simulink model "pd_path_sg"  (R2013b)
settings: Solver=ode45  StartTime=0.0  StopTime=10  RelTol=1e-3
undefined symbols (not defined in the file or in its folder): A, A2, B, C, D, EVAL, i, output_samp_bcoef, PCIN, reg_pk_lim, reg_plim, reg_scale, reg_sr_lim, reg_staclr, reg_txgain, THIS_DATE, W, X, Z
undefined symbols (not defined in the file): lut_address, lut_address_s5, reg_dltap
libraries: xbsIndex_r4 x3819, lut_ram_vhdl x32
(part 27 of 31)

== system pd_path_sg/output_sw_B/config_regs1/perbus_reg3 ==
  addr : Inport
  din : Inport  Port=2
  we : Inport  Port=3
  rst : Inport  Port=4
  Logical1 : xbsIndex_r4/Logical  logical_function=AND  inputs=2  en=off  latency=0  precision=Full  arith_type=Unsigned  n_bits=16  bin_pt=0  align_bp=on  dbl_ovrd=off  block_type=logical
  REG_ADDR : xbsIndex_r4/Constant  const=reg_txgain(para_band+1)  gui_display_data_type=Fixed-point  arith_type=Unsigned  n_bits=12  bin_pt=0  preci_type=Single  exp_width=8  frac_width=24  explicit_period=off  period=1  equ=P=C  opselect=C  inp2=PCIN>>17  opr=+  inp1=P  carry=CIN  dbl_ovrd=off  block_type=constant
  Register : xbsIndex_r4/Register  init=16384  rst=on  en=on  dbl_ovrd=off  block_type=register
  Relational2 : xbsIndex_r4/Relational  mode=a=b  op_type=Bool  en=off  latency=0  dbl_ovrd=off  block_type=relational
  q : Outport
  wires:
  REG_ADDR/1 -> Relational2/2
  Relational2/1 -> Logical1/2
  Logical1/1 -> Register/3
  addr/1 -> Relational2/1
  we/1 -> Logical1/1
  din/1 -> Register/1
  Register/1 -> q/1
  rst/1 -> Register/2

== system pd_path_sg/output_sw_B/detect_i/cut8bit ==
  d : Inport
  Convert : xbsIndex_r4/Convert  gui_display_data_type=Fixed-point  arith_type="Signed  (2's comp)"  n_bits=17  bin_pt=0  float_type=Single  exp_bits=8  fraction_bits=24  quantization=Truncate  overflow=Wrap  en=off  latency=0  pipeline=off  dbl_ovrd=off  block_type=convert
  Reinterpret4 : xbsIndex_r4/Reinterpret  force_arith_type=on  arith_type="Signed  (2's comp)"  force_bin_pt=off  bin_pt=0  block_type=reinterpret
  Slice1 : xbsIndex_r4/Slice  nbits=9  boolean_output=off  mode=Upper Bit Location + Width  bit1=0  base1=MSB of Input  bit0=0  base0=LSB of Input  dbl_ovrd=off  block_type=slice
  q : Outport
  wires:
  Reinterpret4/1 -> q/1
  d/1 -> Convert/1
  Convert/1 -> Slice1/1
  Slice1/1 -> Reinterpret4/1

== system pd_path_sg/output_sw_B/detect_i/cut8bit1 ==
  d : Inport
  Convert : xbsIndex_r4/Convert  gui_display_data_type=Fixed-point  arith_type="Signed  (2's comp)"  n_bits=17  bin_pt=0  float_type=Single  exp_bits=8  fraction_bits=24  quantization=Truncate  overflow=Wrap  en=off  latency=0  pipeline=off  dbl_ovrd=off  block_type=convert
  Reinterpret4 : xbsIndex_r4/Reinterpret  force_arith_type=on  arith_type="Signed  (2's comp)"  force_bin_pt=off  bin_pt=0  block_type=reinterpret
  Slice1 : xbsIndex_r4/Slice  nbits=9  boolean_output=off  mode=Upper Bit Location + Width  bit1=0  base1=MSB of Input  bit0=0  base0=LSB of Input  dbl_ovrd=off  block_type=slice
  q : Outport
  wires:
  Slice1/1 -> Reinterpret4/1
  Convert/1 -> Slice1/1
  d/1 -> Convert/1
  Reinterpret4/1 -> q/1

== system pd_path_sg/output_sw_B/detect_i/cut8bit2 ==
  d : Inport
  Convert : xbsIndex_r4/Convert  gui_display_data_type=Fixed-point  arith_type="Signed  (2's comp)"  n_bits=17  bin_pt=0  float_type=Single  exp_bits=8  fraction_bits=24  quantization=Truncate  overflow=Wrap  en=off  latency=0  pipeline=off  dbl_ovrd=off  block_type=convert
  Reinterpret4 : xbsIndex_r4/Reinterpret  force_arith_type=on  arith_type="Signed  (2's comp)"  force_bin_pt=off  bin_pt=0  block_type=reinterpret
  Slice1 : xbsIndex_r4/Slice  nbits=9  boolean_output=off  mode=Upper Bit Location + Width  bit1=0  base1=MSB of Input  bit0=0  base0=LSB of Input  dbl_ovrd=off  block_type=slice
  q : Outport
  wires:
  Reinterpret4/1 -> q/1
  d/1 -> Convert/1
  Convert/1 -> Slice1/1
  Slice1/1 -> Reinterpret4/1

== system pd_path_sg/output_sw_B/detect_i/cut8bit3 ==
  d : Inport
  Convert : xbsIndex_r4/Convert  gui_display_data_type=Fixed-point  arith_type="Signed  (2's comp)"  n_bits=17  bin_pt=0  float_type=Single  exp_bits=8  fraction_bits=24  quantization=Truncate  overflow=Wrap  en=off  latency=0  pipeline=off  dbl_ovrd=off  block_type=convert
  Reinterpret4 : xbsIndex_r4/Reinterpret  force_arith_type=on  arith_type="Signed  (2's comp)"  force_bin_pt=off  bin_pt=0  block_type=reinterpret
  Slice1 : xbsIndex_r4/Slice  nbits=9  boolean_output=off  mode=Upper Bit Location + Width  bit1=0  base1=MSB of Input  bit0=0  base0=LSB of Input  dbl_ovrd=off  block_type=slice
  q : Outport
  wires:
  Slice1/1 -> Reinterpret4/1
  Convert/1 -> Slice1/1
  d/1 -> Convert/1
  Reinterpret4/1 -> q/1

== system pd_path_sg/output_sw_B/detect_i/cut8bit4 ==
  d : Inport
  Convert : xbsIndex_r4/Convert  gui_display_data_type=Fixed-point  arith_type="Signed  (2's comp)"  n_bits=17  bin_pt=0  float_type=Single  exp_bits=8  fraction_bits=24  quantization=Truncate  overflow=Wrap  en=off  latency=0  pipeline=off  dbl_ovrd=off  block_type=convert
  Reinterpret4 : xbsIndex_r4/Reinterpret  force_arith_type=on  arith_type="Signed  (2's comp)"  force_bin_pt=off  bin_pt=0  block_type=reinterpret
  Slice1 : xbsIndex_r4/Slice  nbits=9  boolean_output=off  mode=Upper Bit Location + Width  bit1=0  base1=MSB of Input  bit0=0  base0=LSB of Input  dbl_ovrd=off  block_type=slice
  q : Outport
  wires:
  Reinterpret4/1 -> q/1
  d/1 -> Convert/1
  Convert/1 -> Slice1/1
  Slice1/1 -> Reinterpret4/1

== system pd_path_sg/output_sw_B/detect_i/cut8bit5 ==
  d : Inport
  Convert : xbsIndex_r4/Convert  gui_display_data_type=Fixed-point  arith_type="Signed  (2's comp)"  n_bits=17  bin_pt=0  float_type=Single  exp_bits=8  fraction_bits=24  quantization=Truncate  overflow=Wrap  en=off  latency=0  pipeline=off  dbl_ovrd=off  block_type=convert
  Reinterpret4 : xbsIndex_r4/Reinterpret  force_arith_type=on  arith_type="Signed  (2's comp)"  force_bin_pt=off  bin_pt=0  block_type=reinterpret
  Slice1 : xbsIndex_r4/Slice  nbits=9  boolean_output=off  mode=Upper Bit Location + Width  bit1=0  base1=MSB of Input  bit0=0  base0=LSB of Input  dbl_ovrd=off  block_type=slice
  q : Outport
  wires:
  Slice1/1 -> Reinterpret4/1
  Convert/1 -> Slice1/1
  d/1 -> Convert/1
  Reinterpret4/1 -> q/1

== system pd_path_sg/output_sw_B/detect_q/cut8bit ==
  d : Inport
  Convert : xbsIndex_r4/Convert  gui_display_data_type=Fixed-point  arith_type="Signed  (2's comp)"  n_bits=17  bin_pt=0  float_type=Single  exp_bits=8  fraction_bits=24  quantization=Truncate  overflow=Wrap  en=off  latency=0  pipeline=off  dbl_ovrd=off  block_type=convert
  Reinterpret4 : xbsIndex_r4/Reinterpret  force_arith_type=on  arith_type="Signed  (2's comp)"  force_bin_pt=off  bin_pt=0  block_type=reinterpret
  Slice1 : xbsIndex_r4/Slice  nbits=9  boolean_output=off  mode=Upper Bit Location + Width  bit1=0  base1=MSB of Input  bit0=0  base0=LSB of Input  dbl_ovrd=off  block_type=slice
  q : Outport
  wires:
  Slice1/1 -> Reinterpret4/1
  Convert/1 -> Slice1/1
  d/1 -> Convert/1
  Reinterpret4/1 -> q/1

== system pd_path_sg/output_sw_B/detect_q/cut8bit1 ==
  d : Inport
  Convert : xbsIndex_r4/Convert  gui_display_data_type=Fixed-point  arith_type="Signed  (2's comp)"  n_bits=17  bin_pt=0  float_type=Single  exp_bits=8  fraction_bits=24  quantization=Truncate  overflow=Wrap  en=off  latency=0  pipeline=off  dbl_ovrd=off  block_type=convert
  Reinterpret4 : xbsIndex_r4/Reinterpret  force_arith_type=on  arith_type="Signed  (2's comp)"  force_bin_pt=off  bin_pt=0  block_type=reinterpret
  Slice1 : xbsIndex_r4/Slice  nbits=9  boolean_output=off  mode=Upper Bit Location + Width  bit1=0  base1=MSB of Input  bit0=0  base0=LSB of Input  dbl_ovrd=off  block_type=slice
  q : Outport
  wires:
  Reinterpret4/1 -> q/1
  d/1 -> Convert/1
  Convert/1 -> Slice1/1
  Slice1/1 -> Reinterpret4/1

== system pd_path_sg/output_sw_B/detect_q/cut8bit2 ==
  d : Inport
  Convert : xbsIndex_r4/Convert  gui_display_data_type=Fixed-point  arith_type="Signed  (2's comp)"  n_bits=17  bin_pt=0  float_type=Single  exp_bits=8  fraction_bits=24  quantization=Truncate  overflow=Wrap  en=off  latency=0  pipeline=off  dbl_ovrd=off  block_type=convert
  Reinterpret4 : xbsIndex_r4/Reinterpret  force_arith_type=on  arith_type="Signed  (2's comp)"  force_bin_pt=off  bin_pt=0  block_type=reinterpret
  Slice1 : xbsIndex_r4/Slice  nbits=9  boolean_output=off  mode=Upper Bit Location + Width  bit1=0  base1=MSB of Input  bit0=0  base0=LSB of Input  dbl_ovrd=off  block_type=slice
  q : Outport
  wires:
  Slice1/1 -> Reinterpret4/1
  Convert/1 -> Slice1/1
  d/1 -> Convert/1
  Reinterpret4/1 -> q/1

== system pd_path_sg/output_sw_B/detect_q/cut8bit3 ==
  d : Inport
  Convert : xbsIndex_r4/Convert  gui_display_data_type=Fixed-point  arith_type="Signed  (2's comp)"  n_bits=17  bin_pt=0  float_type=Single  exp_bits=8  fraction_bits=24  quantization=Truncate  overflow=Wrap  en=off  latency=0  pipeline=off  dbl_ovrd=off  block_type=convert
  Reinterpret4 : xbsIndex_r4/Reinterpret  force_arith_type=on  arith_type="Signed  (2's comp)"  force_bin_pt=off  bin_pt=0  block_type=reinterpret
  Slice1 : xbsIndex_r4/Slice  nbits=9  boolean_output=off  mode=Upper Bit Location + Width  bit1=0  base1=MSB of Input  bit0=0  base0=LSB of Input  dbl_ovrd=off  block_type=slice
  q : Outport
  wires:
  Reinterpret4/1 -> q/1
  d/1 -> Convert/1
  Convert/1 -> Slice1/1
  Slice1/1 -> Reinterpret4/1

== system pd_path_sg/output_sw_B/detect_q/cut8bit4 ==
  d : Inport
  Convert : xbsIndex_r4/Convert  gui_display_data_type=Fixed-point  arith_type="Signed  (2's comp)"  n_bits=17  bin_pt=0  float_type=Single  exp_bits=8  fraction_bits=24  quantization=Truncate  overflow=Wrap  en=off  latency=0  pipeline=off  dbl_ovrd=off  block_type=convert
  Reinterpret4 : xbsIndex_r4/Reinterpret  force_arith_type=on  arith_type="Signed  (2's comp)"  force_bin_pt=off  bin_pt=0  block_type=reinterpret
  Slice1 : xbsIndex_r4/Slice  nbits=9  boolean_output=off  mode=Upper Bit Location + Width  bit1=0  base1=MSB of Input  bit0=0  base0=LSB of Input  dbl_ovrd=off  block_type=slice
  q : Outport
  wires:
  Slice1/1 -> Reinterpret4/1
  Convert/1 -> Slice1/1
  d/1 -> Convert/1
  Reinterpret4/1 -> q/1

== system pd_path_sg/output_sw_B/detect_q/cut8bit5 ==
  d : Inport
  Convert : xbsIndex_r4/Convert  gui_display_data_type=Fixed-point  arith_type="Signed  (2's comp)"  n_bits=17  bin_pt=0  float_type=Single  exp_bits=8  fraction_bits=24  quantization=Truncate  overflow=Wrap  en=off  latency=0  pipeline=off  dbl_ovrd=off  block_type=convert
  Reinterpret4 : xbsIndex_r4/Reinterpret  force_arith_type=on  arith_type="Signed  (2's comp)"  force_bin_pt=off  bin_pt=0  block_type=reinterpret
  Slice1 : xbsIndex_r4/Slice  nbits=9  boolean_output=off  mode=Upper Bit Location + Width  bit1=0  base1=MSB of Input  bit0=0  base0=LSB of Input  dbl_ovrd=off  block_type=slice
  q : Outport
  wires:
  Reinterpret4/1 -> q/1
  d/1 -> Convert/1
  Convert/1 -> Slice1/1
  Slice1/1 -> Reinterpret4/1

== system pd_path_sg/resamp_mod/mod0/imag_modu ==
  Ai : Inport
  Aq : Inport  Port=2
  Bi : Inport  Port=3
  Bq : Inport  Port=4
  sin : Inport  Port=5
  cos : Inport  Port=6
  Constant1 : xbsIndex_r4/Constant  const=2^13  gui_display_data_type=Fixed-point  arith_type=Signed (2's comp)  n_bits=48  bin_pt=0  preci_type=Single  exp_width=8  frac_width=24  explicit_period=off  period=1  equ=P=C  opselect=C  inp2=PCIN>>17  opr=+  inp1=P  carry=CIN  dbl_ovrd=off  block_type=constant
  Convert10 : xbsIndex_r4/Convert  gui_display_data_type=Fixed-point  arith_type="Signed  (2's comp)"  n_bits=18  bin_pt=0  float_type=Single  exp_bits=8  fraction_bits=24  quantization=Truncate  overflow=Wrap  en=off  latency=0  pipeline=off  dbl_ovrd=off  block_type=convert
  Convert11 : xbsIndex_r4/Convert  gui_display_data_type=Fixed-point  arith_type="Signed  (2's comp)"  n_bits=27  bin_pt=0  float_type=Single  exp_bits=8  fraction_bits=24  quantization=Truncate  overflow=Wrap  en=off  latency=0  pipeline=off  dbl_ovrd=off  block_type=convert
  Convert5 : xbsIndex_r4/Convert  gui_display_data_type=Fixed-point  arith_type="Signed  (2's comp)"  n_bits=30  bin_pt=0  float_type=Single  exp_bits=8  fraction_bits=24  quantization=Truncate  overflow=Wrap  en=off  latency=0  pipeline=off  dbl_ovrd=off  block_type=convert
  Convert6 : xbsIndex_r4/Convert  gui_display_data_type=Fixed-point  arith_type="Signed  (2's comp)"  n_bits=18  bin_pt=0  float_type=Single  exp_bits=8  fraction_bits=24  quantization=Truncate  overflow=Wrap  en=off  latency=0  pipeline=off  dbl_ovrd=off  block_type=convert
  Convert8 : xbsIndex_r4/Convert  gui_display_data_type=Fixed-point  arith_type="Signed  (2's comp)"  n_bits=27  bin_pt=0  float_type=Single  exp_bits=8  fraction_bits=24  quantization=Truncate  overflow=Wrap  en=off  latency=0  pipeline=off  dbl_ovrd=off  block_type=convert
  Convert9 : xbsIndex_r4/Convert  gui_display_data_type=Fixed-point  arith_type="Signed  (2's comp)"  n_bits=30  bin_pt=0  float_type=Single  exp_bits=8  fraction_bits=24  quantization=Truncate  overflow=Wrap  en=off  latency=0  pipeline=off  dbl_ovrd=off  block_type=convert
  "DSP48E2 " : xbsIndex_r4/DSP48E2   use_a=Direct from A Port  use_b=Direct from B Port  addsub_mode=ONE48  xl_useadderonly=off  xl_dynamicmult=off  preaddinsel=A  amultsel=AD  bmultsel=B  enable_d=on  reset_preg=off  auto_reset_pr=RESET  pattern_from_creg=1  pattern='000000000000'  mask_from_creg=1  pattern_mask='000000000000'  rnd='000000000000'  widexor=off  xormode=1  use_op=on  use_creg=on  rst_all=off  en_all=off  use_pcin=off  use_carrycascin=off  use_multsignin=off  use_carryout=off  use_patterndetect=off  use_patternbdetect=off  use_overflow=off  use_underflow=off  use_acout=off  use_bcout=off  use_pcout=on  use_multsignout=off  use_carrycascout=off  pipeline_a=1  pipeline_b=2  pipeline_acout=1  pipeline_bcout=1  pipeline_c=on  pipeline_p=on  pipeline_mult=on  pipeline_opmode=on  pipeline_alumode=on  pipeline_carryin=on  pipeline_carryinsel=on  dreg=on  adreg=on  register_inmode=on  rst_a=off  rst_b=off  rst_c=off  rst_mult=off  rst_p=off  rst_carry_in=off  rst_alumode=off  rst_ctrl=off  reset_port_d=off  reset_port_inmode=off  en_a1=off  en_a2=off  en_b1=off  en_b2=off  en_c=off  en_mult=off  en_p=off  en_carry_in=off  en_alumode=off  en_multcarryin=off  en_ctrl=off  enable_port_regd=off  enable_port_regad=off  enable_port_reginmode=off  alumode_inverted=off  alumode_inverted_value='0000'  is_carryin_inverted=off  inmode_inverted=off  inmode_inverted_value='00000'  opmode_inverted=off  opmode_inverted_value='000000000'  is_rstallcarryin_inverted=off  is_rstalumode_inverted=off  is_rsta_inverted=off  is_rstb_inverted=off  is_rstc_inverted=off  is_rstd_inverted=off  is_rstctrl_inverted=off  is_rstinmode_inverted=off  is_rstm_inverted=off  is_rstp_inverted=off  use_synth_model=off  is_clk_inverted=false  block_type=dsp48e2
  DSP48E2 1 : xbsIndex_r4/DSP48E2   use_a=Direct from A Port  use_b=Direct from B Port  addsub_mode=ONE48  xl_useadderonly=off  xl_dynamicmult=off  preaddinsel=A  amultsel=AD  bmultsel=B  enable_d=on  reset_preg=off  auto_reset_pr=RESET  pattern_from_creg=1  pattern='000000000000'  mask_from_creg=1  pattern_mask='000000000000'  rnd='000000000000'  widexor=off  xormode=1  use_op=on  use_creg=off  rst_all=off  en_all=off  use_pcin=on  use_carrycascin=off  use_multsignin=off  use_carryout=off  use_patterndetect=off  use_patternbdetect=off  use_overflow=off  use_underflow=off  use_acout=off  use_bcout=off  use_pcout=off  use_multsignout=off  use_carrycascout=off  pipeline_a=2  pipeline_b=2  pipeline_acout=1  pipeline_bcout=1  pipeline_c=on  pipeline_p=on  pipeline_mult=on  pipeline_opmode=on  pipeline_alumode=on  pipeline_carryin=on  pipeline_carryinsel=on  dreg=on  adreg=on  register_inmode=on  rst_a=off  rst_b=off  rst_c=off  rst_mult=off  rst_p=off  rst_carry_in=off  rst_alumode=off  rst_ctrl=off  reset_port_d=off  reset_port_inmode=off  en_a1=off  en_a2=off  en_b1=off  en_b2=off  en_c=off  en_mult=off  en_p=off  en_carry_in=off  en_alumode=off  en_multcarryin=off  en_ctrl=off  enable_port_regd=off  enable_port_regad=off  enable_port_reginmode=off  alumode_inverted=off  alumode_inverted_value='0000'  is_carryin_inverted=off  inmode_inverted=off  inmode_inverted_value='00000'  opmode_inverted=off  opmode_inverted_value='000000000'  is_rstallcarryin_inverted=off  is_rstalumode_inverted=off  is_rsta_inverted=off  is_rstb_inverted=off  is_rstc_inverted=off  is_rstd_inverted=off  is_rstctrl_inverted=off  is_rstinmode_inverted=off  is_rstm_inverted=off  is_rstp_inverted=off  use_synth_model=off  is_clk_inverted=false  block_type=dsp48e2
  Delay : xbsIndex_r4/Delay  rst=off  infoeditControl=Selection of Reset will increase slice count due to use of real FFs and instead of SRLs  en=off  latency=1  reg_retiming=off  dbl_ovrd=off  block_type=delay
      settings: infoedit=Hardware notes: A delay line is a chain, each link of which is an SRL16 or SRL32 followed by a flip-flop.
  Delay1 : xbsIndex_r4/Delay  rst=off  infoeditControl=Selection of Reset will increase slice count due to use of real FFs and instead of SRLs  en=off  latency=1  reg_retiming=off  dbl_ovrd=off  block_type=delay
      settings: infoedit=Hardware notes: A delay line is a chain, each link of which is an SRL16 or SRL32 followed by a flip-flop.
  Opmode1 : xbsIndex_r4/Opmode  device=DSP48E2  equ=P=C+(A*B)  operation=Custom  inmode_0_3=D+A2  inmode_1_3=(D+A)*B  preaddinsel=A  amultsel=AD  bmultsel=B  inmode_0=A2  inmode_4=B2  logicinstr=X + W + Z  z_mux=C  xy_mux=A*B  w_mux=0  carry=0  dbl_ovrd=off  operand=+  x_mux=P  block_type=opmode
  Opmode4 : xbsIndex_r4/Opmode  device=DSP48E2  equ=P=PCIN+(A*B)  operation=Custom  inmode_0_3=D+A2  inmode_1_3=(D-A)*B  preaddinsel=A  amultsel=AD  bmultsel=B  inmode_0=A2  inmode_4=B2  logicinstr=X + W + Z  z_mux=PCIN  xy_mux=A*B  w_mux=0  carry=0  dbl_ovrd=off  operand=+  x_mux=P  block_type=opmode
  Reinterpret{5..10,13} (7 alike) : xbsIndex_r4/Reinterpret  force_arith_type=on  arith_type="Signed  (2's comp)"  force_bin_pt=on  bin_pt=0  block_type=reinterpret
  Terminator1 : Terminator
  round1 : Subsystem
  out_imag : Outport
  wires:
  Convert11/1 -> Delay/1
  Convert10/1 -> Delay1/1
  Reinterpret9/1 -> Convert10/1
  Reinterpret10/1 -> Convert11/1
  Reinterpret8/1 -> Convert9/1
  Constant1/1 -> "DSP48E2 "/3
  Bq/1 -> Reinterpret7/1
  Convert9/1 -> DSP48E2 1/1
  sin/1 -> Reinterpret9/1
  Reinterpret7/1 -> Convert8/1
  Aq/1 -> Reinterpret5/1
  cos/1 -> Reinterpret6/1
  Convert6/1 -> "DSP48E2 "/2
  Convert8/1 -> "DSP48E2 "/4
  Ai/1 -> Reinterpret10/1
  Bi/1 -> Reinterpret8/1
  "DSP48E2 "/1 -> Terminator1/1
  DSP48E2 1/1 -> Reinterpret13/1
  Convert5/1 -> "DSP48E2 "/1
  Reinterpret6/1 -> Convert6/1
  "DSP48E2 "/2 -> DSP48E2 1/3
  Reinterpret5/1 -> Convert5/1
  Reinterpret13/1 -> round1/1(d)
  round1/1(q) -> out_imag/1
  Delay/1 -> DSP48E2 1/4
  Delay1/1 -> DSP48E2 1/2
  Opmode1/1 -> "DSP48E2 "/5
  Opmode4/1 -> DSP48E2 1/5

== system pd_path_sg/resamp_mod/mod0/real_modu ==
  Ai : Inport
  Aq : Inport  Port=2
  Bi : Inport  Port=3
  Bq : Inport  Port=4
  sin : Inport  Port=5
  cos : Inport  Port=6
  Constant3 : xbsIndex_r4/Constant  const=2^13  gui_display_data_type=Fixed-point  arith_type=Signed (2's comp)  n_bits=48  bin_pt=0  preci_type=Single  exp_width=8  frac_width=24  explicit_period=off  period=1  equ=P=C  opselect=C  inp2=PCIN>>17  opr=+  inp1=P  carry=CIN  dbl_ovrd=off  block_type=constant
  Convert : xbsIndex_r4/Convert  gui_display_data_type=Fixed-point  arith_type="Signed  (2's comp)"  n_bits=30  bin_pt=0  float_type=Single  exp_bits=8  fraction_bits=24  quantization=Truncate  overflow=Wrap  en=off  latency=0  pipeline=off  dbl_ovrd=off  block_type=convert
  Convert1 : xbsIndex_r4/Convert  gui_display_data_type=Fixed-point  arith_type="Signed  (2's comp)"  n_bits=18  bin_pt=0  float_type=Single  exp_bits=8  fraction_bits=24  quantization=Truncate  overflow=Wrap  en=off  latency=0  pipeline=off  dbl_ovrd=off  block_type=convert
  Convert2 : xbsIndex_r4/Convert  gui_display_data_type=Fixed-point  arith_type="Signed  (2's comp)"  n_bits=18  bin_pt=0  float_type=Single  exp_bits=8  fraction_bits=24  quantization=Truncate  overflow=Wrap  en=off  latency=0  pipeline=off  dbl_ovrd=off  block_type=convert
  Convert3 : xbsIndex_r4/Convert  gui_display_data_type=Fixed-point  arith_type="Signed  (2's comp)"  n_bits=30  bin_pt=0  float_type=Single  exp_bits=8  fraction_bits=24  quantization=Truncate  overflow=Wrap  en=off  latency=0  pipeline=off  dbl_ovrd=off  block_type=convert
  Convert4 : xbsIndex_r4/Convert  gui_display_data_type=Fixed-point  arith_type="Signed  (2's comp)"  n_bits=27  bin_pt=0  float_type=Single  exp_bits=8  fraction_bits=24  quantization=Truncate  overflow=Wrap  en=off  latency=0  pipeline=off  dbl_ovrd=off  block_type=convert
  Convert7 : xbsIndex_r4/Convert  gui_display_data_type=Fixed-point  arith_type="Signed  (2's comp)"  n_bits=27  bin_pt=0  float_type=Single  exp_bits=8  fraction_bits=24  quantization=Truncate  overflow=Wrap  en=off  latency=0  pipeline=off  dbl_ovrd=off  block_type=convert
  "DSP48E2 " : xbsIndex_r4/DSP48E2   use_a=Direct from A Port  use_b=Direct from B Port  addsub_mode=ONE48  xl_useadderonly=off  xl_dynamicmult=off  preaddinsel=A  amultsel=AD  bmultsel=B  enable_d=on  reset_preg=off  auto_reset_pr=RESET  pattern_from_creg=1  pattern='000000000000'  mask_from_creg=1  pattern_mask='000000000000'  rnd='000000000000'  widexor=off  xormode=1  use_op=on  use_creg=on  rst_all=off  en_all=off  use_pcin=off  use_carrycascin=off  use_multsignin=off  use_carryout=off  use_patterndetect=off  use_patternbdetect=off  use_overflow=off  use_underflow=off  use_acout=off  use_bcout=off  use_pcout=on  use_multsignout=off  use_carrycascout=off  pipeline_a=1  pipeline_b=2  pipeline_acout=1  pipeline_bcout=1  pipeline_c=on  pipeline_p=on  pipeline_mult=on  pipeline_opmode=on  pipeline_alumode=on  pipeline_carryin=on  pipeline_carryinsel=on  dreg=on  adreg=on  register_inmode=on  rst_a=off  rst_b=off  rst_c=off  rst_mult=off  rst_p=off  rst_carry_in=off  rst_alumode=off  rst_ctrl=off  reset_port_d=off  reset_port_inmode=off  en_a1=off  en_a2=off  en_b1=off  en_b2=off  en_c=off  en_mult=off  en_p=off  en_carry_in=off  en_alumode=off  en_multcarryin=off  en_ctrl=off  enable_port_regd=off  enable_port_regad=off  enable_port_reginmode=off  alumode_inverted=off  alumode_inverted_value='0000'  is_carryin_inverted=off  inmode_inverted=off  inmode_inverted_value='00000'  opmode_inverted=off  opmode_inverted_value='000000000'  is_rstallcarryin_inverted=off  is_rstalumode_inverted=off  is_rsta_inverted=off  is_rstb_inverted=off  is_rstc_inverted=off  is_rstd_inverted=off  is_rstctrl_inverted=off  is_rstinmode_inverted=off  is_rstm_inverted=off  is_rstp_inverted=off  use_synth_model=off  is_clk_inverted=false  block_type=dsp48e2
  DSP48E2 1 : xbsIndex_r4/DSP48E2   use_a=Direct from A Port  use_b=Direct from B Port  addsub_mode=ONE48  xl_useadderonly=off  xl_dynamicmult=off  preaddinsel=A  amultsel=AD  bmultsel=B  enable_d=on  reset_preg=off  auto_reset_pr=RESET  pattern_from_creg=1  pattern='000000000000'  mask_from_creg=1  pattern_mask='000000000000'  rnd='000000000000'  widexor=off  xormode=1  use_op=on  use_creg=off  rst_all=off  en_all=off  use_pcin=on  use_carrycascin=off  use_multsignin=off  use_carryout=off  use_patterndetect=off  use_patternbdetect=off  use_overflow=off  use_underflow=off  use_acout=off  use_bcout=off  use_pcout=off  use_multsignout=off  use_carrycascout=off  pipeline_a=2  pipeline_b=2  pipeline_acout=1  pipeline_bcout=1  pipeline_c=on  pipeline_p=on  pipeline_mult=on  pipeline_opmode=on  pipeline_alumode=on  pipeline_carryin=on  pipeline_carryinsel=on  dreg=on  adreg=on  register_inmode=on  rst_a=off  rst_b=off  rst_c=off  rst_mult=off  rst_p=off  rst_carry_in=off  rst_alumode=off  rst_ctrl=off  reset_port_d=off  reset_port_inmode=off  en_a1=off  en_a2=off  en_b1=off  en_b2=off  en_c=off  en_mult=off  en_p=off  en_carry_in=off  en_alumode=off  en_multcarryin=off  en_ctrl=off  enable_port_regd=off  enable_port_regad=off  enable_port_reginmode=off  alumode_inverted=off  alumode_inverted_value='0000'  is_carryin_inverted=off  inmode_inverted=off  inmode_inverted_value='00000'  opmode_inverted=off  opmode_inverted_value='000000000'  is_rstallcarryin_inverted=off  is_rstalumode_inverted=off  is_rsta_inverted=off  is_rstb_inverted=off  is_rstc_inverted=off  is_rstd_inverted=off  is_rstctrl_inverted=off  is_rstinmode_inverted=off  is_rstm_inverted=off  is_rstp_inverted=off  use_synth_model=off  is_clk_inverted=false  block_type=dsp48e2
  Delay : xbsIndex_r4/Delay  rst=off  infoeditControl=Selection of Reset will increase slice count due to use of real FFs and instead of SRLs  en=off  latency=1  reg_retiming=off  dbl_ovrd=off  block_type=delay
      settings: infoedit=Hardware notes: A delay line is a chain, each link of which is an SRL16 or SRL32 followed by a flip-flop.
  Delay1 : xbsIndex_r4/Delay  rst=off  infoeditControl=Selection of Reset will increase slice count due to use of real FFs and instead of SRLs  en=off  latency=1  reg_retiming=off  dbl_ovrd=off  block_type=delay
      settings: infoedit=Hardware notes: A delay line is a chain, each link of which is an SRL16 or SRL32 followed by a flip-flop.
  Opmode2 : xbsIndex_r4/Opmode  device=DSP48E2  equ=P=C+(A*B)  operation=Custom  inmode_0_3=D+A2  inmode_1_3=(D+A)*B  preaddinsel=A  amultsel=AD  bmultsel=B  inmode_0=A2  inmode_4=B2  logicinstr=X + W + Z  z_mux=C  xy_mux=A*B  w_mux=0  carry=0  dbl_ovrd=off  operand=+  x_mux=P  block_type=opmode
  Opmode3 : xbsIndex_r4/Opmode  device=DSP48E2  equ=P=PCIN+(A*B)  operation=Custom  inmode_0_3=D+A2  inmode_1_3=(D-A)*B  preaddinsel=A  amultsel=AD  bmultsel=B  inmode_0=A2  inmode_4=B2  logicinstr=X + W + Z  z_mux=PCIN  xy_mux=A*B  w_mux=0  carry=0  dbl_ovrd=off  operand=+  x_mux=P  block_type=opmode
  Reinterpret{,1..4,11,13} (7 alike) : xbsIndex_r4/Reinterpret  force_arith_type=on  arith_type="Signed  (2's comp)"  force_bin_pt=on  bin_pt=0  block_type=reinterpret
  Terminator : Terminator
  round1 : Subsystem
  out_real : Outport
  wires:
  sin/1 -> Reinterpret1/1
  Aq/1 -> Reinterpret2/1
  Ai/1 -> Reinterpret4/1
  Bq/1 -> Reinterpret3/1
  cos/1 -> Reinterpret/1
  Bi/1 -> Reinterpret11/1
  "DSP48E2 "/2 -> DSP48E2 1/3
  "DSP48E2 "/1 -> Terminator/1
  DSP48E2 1/1 -> Reinterpret13/1
  Reinterpret4/1 -> Convert/1
  Convert1/1 -> "DSP48E2 "/2
  Convert/1 -> "DSP48E2 "/1
  Reinterpret/1 -> Convert1/1
  Convert4/1 -> Delay/1
  Convert2/1 -> Delay1/1
  Convert3/1 -> DSP48E2 1/1
  Reinterpret3/1 -> Convert4/1
  Reinterpret11/1 -> Convert7/1
  Constant3/1 -> "DSP48E2 "/3
  Reinterpret1/1 -> Convert2/1
  Convert7/1 -> "DSP48E2 "/4
  Reinterpret2/1 -> Convert3/1
  Reinterpret13/1 -> round1/1(d)
  round1/1(q) -> out_real/1
  Delay/1 -> DSP48E2 1/4
  Delay1/1 -> DSP48E2 1/2
  Opmode2/1 -> "DSP48E2 "/5
  Opmode3/1 -> DSP48E2 1/5

== system pd_path_sg/resamp_mod/mod1/imag_modu ==
  Ai : Inport
  Aq : Inport  Port=2
  Bi : Inport  Port=3
  Bq : Inport  Port=4
  sin : Inport  Port=5
  cos : Inport  Port=6
  Constant1 : xbsIndex_r4/Constant  const=2^13  gui_display_data_type=Fixed-point  arith_type=Signed (2's comp)  n_bits=48  bin_pt=0  preci_type=Single  exp_width=8  frac_width=24  explicit_period=off  period=1  equ=P=C  opselect=C  inp2=PCIN>>17  opr=+  inp1=P  carry=CIN  dbl_ovrd=off  block_type=constant
  Convert10 : xbsIndex_r4/Convert  gui_display_data_type=Fixed-point  arith_type="Signed  (2's comp)"  n_bits=18  bin_pt=0  float_type=Single  exp_bits=8  fraction_bits=24  quantization=Truncate  overflow=Wrap  en=off  latency=0  pipeline=off  dbl_ovrd=off  block_type=convert
  Convert11 : xbsIndex_r4/Convert  gui_display_data_type=Fixed-point  arith_type="Signed  (2's comp)"  n_bits=27  bin_pt=0  float_type=Single  exp_bits=8  fraction_bits=24  quantization=Truncate  overflow=Wrap  en=off  latency=0  pipeline=off  dbl_ovrd=off  block_type=convert
  Convert5 : xbsIndex_r4/Convert  gui_display_data_type=Fixed-point  arith_type="Signed  (2's comp)"  n_bits=30  bin_pt=0  float_type=Single  exp_bits=8  fraction_bits=24  quantization=Truncate  overflow=Wrap  en=off  latency=0  pipeline=off  dbl_ovrd=off  block_type=convert
  Convert6 : xbsIndex_r4/Convert  gui_display_data_type=Fixed-point  arith_type="Signed  (2's comp)"  n_bits=18  bin_pt=0  float_type=Single  exp_bits=8  fraction_bits=24  quantization=Truncate  overflow=Wrap  en=off  latency=0  pipeline=off  dbl_ovrd=off  block_type=convert
  Convert8 : xbsIndex_r4/Convert  gui_display_data_type=Fixed-point  arith_type="Signed  (2's comp)"  n_bits=27  bin_pt=0  float_type=Single  exp_bits=8  fraction_bits=24  quantization=Truncate  overflow=Wrap  en=off  latency=0  pipeline=off  dbl_ovrd=off  block_type=convert
  Convert9 : xbsIndex_r4/Convert  gui_display_data_type=Fixed-point  arith_type="Signed  (2's comp)"  n_bits=30  bin_pt=0  float_type=Single  exp_bits=8  fraction_bits=24  quantization=Truncate  overflow=Wrap  en=off  latency=0  pipeline=off  dbl_ovrd=off  block_type=convert
  "DSP48E2 " : xbsIndex_r4/DSP48E2   use_a=Direct from A Port  use_b=Direct from B Port  addsub_mode=ONE48  xl_useadderonly=off  xl_dynamicmult=off  preaddinsel=A  amultsel=AD  bmultsel=B  enable_d=on  reset_preg=off  auto_reset_pr=RESET  pattern_from_creg=1  pattern='000000000000'  mask_from_creg=1  pattern_mask='000000000000'  rnd='000000000000'  widexor=off  xormode=1  use_op=on  use_creg=on  rst_all=off  en_all=off  use_pcin=off  use_carrycascin=off  use_multsignin=off  use_carryout=off  use_patterndetect=off  use_patternbdetect=off  use_overflow=off  use_underflow=off  use_acout=off  use_bcout=off  use_pcout=on  use_multsignout=off  use_carrycascout=off  pipeline_a=1  pipeline_b=2  pipeline_acout=1  pipeline_bcout=1  pipeline_c=on  pipeline_p=on  pipeline_mult=on  pipeline_opmode=on  pipeline_alumode=on  pipeline_carryin=on  pipeline_carryinsel=on  dreg=on  adreg=on  register_inmode=on  rst_a=off  rst_b=off  rst_c=off  rst_mult=off  rst_p=off  rst_carry_in=off  rst_alumode=off  rst_ctrl=off  reset_port_d=off  reset_port_inmode=off  en_a1=off  en_a2=off  en_b1=off  en_b2=off  en_c=off  en_mult=off  en_p=off  en_carry_in=off  en_alumode=off  en_multcarryin=off  en_ctrl=off  enable_port_regd=off  enable_port_regad=off  enable_port_reginmode=off  alumode_inverted=off  alumode_inverted_value='0000'  is_carryin_inverted=off  inmode_inverted=off  inmode_inverted_value='00000'  opmode_inverted=off  opmode_inverted_value='000000000'  is_rstallcarryin_inverted=off  is_rstalumode_inverted=off  is_rsta_inverted=off  is_rstb_inverted=off  is_rstc_inverted=off  is_rstd_inverted=off  is_rstctrl_inverted=off  is_rstinmode_inverted=off  is_rstm_inverted=off  is_rstp_inverted=off  use_synth_model=off  is_clk_inverted=false  block_type=dsp48e2
  DSP48E2 1 : xbsIndex_r4/DSP48E2   use_a=Direct from A Port  use_b=Direct from B Port  addsub_mode=ONE48  xl_useadderonly=off  xl_dynamicmult=off  preaddinsel=A  amultsel=AD  bmultsel=B  enable_d=on  reset_preg=off  auto_reset_pr=RESET  pattern_from_creg=1  pattern='000000000000'  mask_from_creg=1  pattern_mask='000000000000'  rnd='000000000000'  widexor=off  xormode=1  use_op=on  use_creg=off  rst_all=off  en_all=off  use_pcin=on  use_carrycascin=off  use_multsignin=off  use_carryout=off  use_patterndetect=off  use_patternbdetect=off  use_overflow=off  use_underflow=off  use_acout=off  use_bcout=off  use_pcout=off  use_multsignout=off  use_carrycascout=off  pipeline_a=2  pipeline_b=2  pipeline_acout=1  pipeline_bcout=1  pipeline_c=on  pipeline_p=on  pipeline_mult=on  pipeline_opmode=on  pipeline_alumode=on  pipeline_carryin=on  pipeline_carryinsel=on  dreg=on  adreg=on  register_inmode=on  rst_a=off  rst_b=off  rst_c=off  rst_mult=off  rst_p=off  rst_carry_in=off  rst_alumode=off  rst_ctrl=off  reset_port_d=off  reset_port_inmode=off  en_a1=off  en_a2=off  en_b1=off  en_b2=off  en_c=off  en_mult=off  en_p=off  en_carry_in=off  en_alumode=off  en_multcarryin=off  en_ctrl=off  enable_port_regd=off  enable_port_regad=off  enable_port_reginmode=off  alumode_inverted=off  alumode_inverted_value='0000'  is_carryin_inverted=off  inmode_inverted=off  inmode_inverted_value='00000'  opmode_inverted=off  opmode_inverted_value='000000000'  is_rstallcarryin_inverted=off  is_rstalumode_inverted=off  is_rsta_inverted=off  is_rstb_inverted=off  is_rstc_inverted=off  is_rstd_inverted=off  is_rstctrl_inverted=off  is_rstinmode_inverted=off  is_rstm_inverted=off  is_rstp_inverted=off  use_synth_model=off  is_clk_inverted=false  block_type=dsp48e2
  Delay : xbsIndex_r4/Delay  rst=off  infoeditControl=Selection of Reset will increase slice count due to use of real FFs and instead of SRLs  en=off  latency=1  reg_retiming=off  dbl_ovrd=off  block_type=delay
      settings: infoedit=Hardware notes: A delay line is a chain, each link of which is an SRL16 or SRL32 followed by a flip-flop.
  Delay1 : xbsIndex_r4/Delay  rst=off  infoeditControl=Selection of Reset will increase slice count due to use of real FFs and instead of SRLs  en=off  latency=1  reg_retiming=off  dbl_ovrd=off  block_type=delay
      settings: infoedit=Hardware notes: A delay line is a chain, each link of which is an SRL16 or SRL32 followed by a flip-flop.
  Opmode1 : xbsIndex_r4/Opmode  device=DSP48E2  equ=P=C+(A*B)  operation=Custom  inmode_0_3=D+A2  inmode_1_3=(D+A)*B  preaddinsel=A  amultsel=AD  bmultsel=B  inmode_0=A2  inmode_4=B2  logicinstr=X + W + Z  z_mux=C  xy_mux=A*B  w_mux=0  carry=0  dbl_ovrd=off  operand=+  x_mux=P  block_type=opmode
  Opmode4 : xbsIndex_r4/Opmode  device=DSP48E2  equ=P=PCIN+(A*B)  operation=Custom  inmode_0_3=D+A2  inmode_1_3=(D-A)*B  preaddinsel=A  amultsel=AD  bmultsel=B  inmode_0=A2  inmode_4=B2  logicinstr=X + W + Z  z_mux=PCIN  xy_mux=A*B  w_mux=0  carry=0  dbl_ovrd=off  operand=+  x_mux=P  block_type=opmode
  Reinterpret{5..10,13} (7 alike) : xbsIndex_r4/Reinterpret  force_arith_type=on  arith_type="Signed  (2's comp)"  force_bin_pt=on  bin_pt=0  block_type=reinterpret
  Terminator1 : Terminator
  round1 : Subsystem
  out_imag : Outport
  wires:
  Opmode4/1 -> DSP48E2 1/5
  Opmode1/1 -> "DSP48E2 "/5
  Delay1/1 -> DSP48E2 1/2
  Delay/1 -> DSP48E2 1/4
  round1/1(q) -> out_imag/1
  Reinterpret13/1 -> round1/1(d)
  Reinterpret5/1 -> Convert5/1
  "DSP48E2 "/2 -> DSP48E2 1/3
  Reinterpret6/1 -> Convert6/1
  Convert5/1 -> "DSP48E2 "/1
  DSP48E2 1/1 -> Reinterpret13/1
  "DSP48E2 "/1 -> Terminator1/1
  Bi/1 -> Reinterpret8/1
  Ai/1 -> Reinterpret10/1
  Convert8/1 -> "DSP48E2 "/4
  Convert6/1 -> "DSP48E2 "/2
  cos/1 -> Reinterpret6/1
  Aq/1 -> Reinterpret5/1
  Reinterpret7/1 -> Convert8/1
  sin/1 -> Reinterpret9/1
  Convert9/1 -> DSP48E2 1/1
  Bq/1 -> Reinterpret7/1
  Constant1/1 -> "DSP48E2 "/3
  Reinterpret8/1 -> Convert9/1
  Reinterpret10/1 -> Convert11/1
  Reinterpret9/1 -> Convert10/1
  Convert10/1 -> Delay1/1
  Convert11/1 -> Delay/1

== system pd_path_sg/resamp_mod/mod1/real_modu ==
  Ai : Inport
  Aq : Inport  Port=2
  Bi : Inport  Port=3
  Bq : Inport  Port=4
  sin : Inport  Port=5
  cos : Inport  Port=6
  Constant3 : xbsIndex_r4/Constant  const=2^13  gui_display_data_type=Fixed-point  arith_type=Signed (2's comp)  n_bits=48  bin_pt=0  preci_type=Single  exp_width=8  frac_width=24  explicit_period=off  period=1  equ=P=C  opselect=C  inp2=PCIN>>17  opr=+  inp1=P  carry=CIN  dbl_ovrd=off  block_type=constant
  Convert : xbsIndex_r4/Convert  gui_display_data_type=Fixed-point  arith_type="Signed  (2's comp)"  n_bits=30  bin_pt=0  float_type=Single  exp_bits=8  fraction_bits=24  quantization=Truncate  overflow=Wrap  en=off  latency=0  pipeline=off  dbl_ovrd=off  block_type=convert
  Convert1 : xbsIndex_r4/Convert  gui_display_data_type=Fixed-point  arith_type="Signed  (2's comp)"  n_bits=18  bin_pt=0  float_type=Single  exp_bits=8  fraction_bits=24  quantization=Truncate  overflow=Wrap  en=off  latency=0  pipeline=off  dbl_ovrd=off  block_type=convert
  Convert2 : xbsIndex_r4/Convert  gui_display_data_type=Fixed-point  arith_type="Signed  (2's comp)"  n_bits=18  bin_pt=0  float_type=Single  exp_bits=8  fraction_bits=24  quantization=Truncate  overflow=Wrap  en=off  latency=0  pipeline=off  dbl_ovrd=off  block_type=convert
  Convert3 : xbsIndex_r4/Convert  gui_display_data_type=Fixed-point  arith_type="Signed  (2's comp)"  n_bits=30  bin_pt=0  float_type=Single  exp_bits=8  fraction_bits=24  quantization=Truncate  overflow=Wrap  en=off  latency=0  pipeline=off  dbl_ovrd=off  block_type=convert
  Convert4 : xbsIndex_r4/Convert  gui_display_data_type=Fixed-point  arith_type="Signed  (2's comp)"  n_bits=27  bin_pt=0  float_type=Single  exp_bits=8  fraction_bits=24  quantization=Truncate  overflow=Wrap  en=off  latency=0  pipeline=off  dbl_ovrd=off  block_type=convert
  Convert7 : xbsIndex_r4/Convert  gui_display_data_type=Fixed-point  arith_type="Signed  (2's comp)"  n_bits=27  bin_pt=0  float_type=Single  exp_bits=8  fraction_bits=24  quantization=Truncate  overflow=Wrap  en=off  latency=0  pipeline=off  dbl_ovrd=off  block_type=convert
  "DSP48E2 " : xbsIndex_r4/DSP48E2   use_a=Direct from A Port  use_b=Direct from B Port  addsub_mode=ONE48  xl_useadderonly=off  xl_dynamicmult=off  preaddinsel=A  amultsel=AD  bmultsel=B  enable_d=on  reset_preg=off  auto_reset_pr=RESET  pattern_from_creg=1  pattern='000000000000'  mask_from_creg=1  pattern_mask='000000000000'  rnd='000000000000'  widexor=off  xormode=1  use_op=on  use_creg=on  rst_all=off  en_all=off  use_pcin=off  use_carrycascin=off  use_multsignin=off  use_carryout=off  use_patterndetect=off  use_patternbdetect=off  use_overflow=off  use_underflow=off  use_acout=off  use_bcout=off  use_pcout=on  use_multsignout=off  use_carrycascout=off  pipeline_a=1  pipeline_b=2  pipeline_acout=1  pipeline_bcout=1  pipeline_c=on  pipeline_p=on  pipeline_mult=on  pipeline_opmode=on  pipeline_alumode=on  pipeline_carryin=on  pipeline_carryinsel=on  dreg=on  adreg=on  register_inmode=on  rst_a=off  rst_b=off  rst_c=off  rst_mult=off  rst_p=off  rst_carry_in=off  rst_alumode=off  rst_ctrl=off  reset_port_d=off  reset_port_inmode=off  en_a1=off  en_a2=off  en_b1=off  en_b2=off  en_c=off  en_mult=off  en_p=off  en_carry_in=off  en_alumode=off  en_multcarryin=off  en_ctrl=off  enable_port_regd=off  enable_port_regad=off  enable_port_reginmode=off  alumode_inverted=off  alumode_inverted_value='0000'  is_carryin_inverted=off  inmode_inverted=off  inmode_inverted_value='00000'  opmode_inverted=off  opmode_inverted_value='000000000'  is_rstallcarryin_inverted=off  is_rstalumode_inverted=off  is_rsta_inverted=off  is_rstb_inverted=off  is_rstc_inverted=off  is_rstd_inverted=off  is_rstctrl_inverted=off  is_rstinmode_inverted=off  is_rstm_inverted=off  is_rstp_inverted=off  use_synth_model=off  is_clk_inverted=false  block_type=dsp48e2
  DSP48E2 1 : xbsIndex_r4/DSP48E2   use_a=Direct from A Port  use_b=Direct from B Port  addsub_mode=ONE48  xl_useadderonly=off  xl_dynamicmult=off  preaddinsel=A  amultsel=AD  bmultsel=B  enable_d=on  reset_preg=off  auto_reset_pr=RESET  pattern_from_creg=1  pattern='000000000000'  mask_from_creg=1  pattern_mask='000000000000'  rnd='000000000000'  widexor=off  xormode=1  use_op=on  use_creg=off  rst_all=off  en_all=off  use_pcin=on  use_carrycascin=off  use_multsignin=off  use_carryout=off  use_patterndetect=off  use_patternbdetect=off  use_overflow=off  use_underflow=off  use_acout=off  use_bcout=off  use_pcout=off  use_multsignout=off  use_carrycascout=off  pipeline_a=2  pipeline_b=2  pipeline_acout=1  pipeline_bcout=1  pipeline_c=on  pipeline_p=on  pipeline_mult=on  pipeline_opmode=on  pipeline_alumode=on  pipeline_carryin=on  pipeline_carryinsel=on  dreg=on  adreg=on  register_inmode=on  rst_a=off  rst_b=off  rst_c=off  rst_mult=off  rst_p=off  rst_carry_in=off  rst_alumode=off  rst_ctrl=off  reset_port_d=off  reset_port_inmode=off  en_a1=off  en_a2=off  en_b1=off  en_b2=off  en_c=off  en_mult=off  en_p=off  en_carry_in=off  en_alumode=off  en_multcarryin=off  en_ctrl=off  enable_port_regd=off  enable_port_regad=off  enable_port_reginmode=off  alumode_inverted=off  alumode_inverted_value='0000'  is_carryin_inverted=off  inmode_inverted=off  inmode_inverted_value='00000'  opmode_inverted=off  opmode_inverted_value='000000000'  is_rstallcarryin_inverted=off  is_rstalumode_inverted=off  is_rsta_inverted=off  is_rstb_inverted=off  is_rstc_inverted=off  is_rstd_inverted=off  is_rstctrl_inverted=off  is_rstinmode_inverted=off  is_rstm_inverted=off  is_rstp_inverted=off  use_synth_model=off  is_clk_inverted=false  block_type=dsp48e2
  Delay : xbsIndex_r4/Delay  rst=off  infoeditControl=Selection of Reset will increase slice count due to use of real FFs and instead of SRLs  en=off  latency=1  reg_retiming=off  dbl_ovrd=off  block_type=delay
      settings: infoedit=Hardware notes: A delay line is a chain, each link of which is an SRL16 or SRL32 followed by a flip-flop.
  Delay1 : xbsIndex_r4/Delay  rst=off  infoeditControl=Selection of Reset will increase slice count due to use of real FFs and instead of SRLs  en=off  latency=1  reg_retiming=off  dbl_ovrd=off  block_type=delay
      settings: infoedit=Hardware notes: A delay line is a chain, each link of which is an SRL16 or SRL32 followed by a flip-flop.
  Opmode2 : xbsIndex_r4/Opmode  device=DSP48E2  equ=P=C+(A*B)  operation=Custom  inmode_0_3=D+A2  inmode_1_3=(D+A)*B  preaddinsel=A  amultsel=AD  bmultsel=B  inmode_0=A2  inmode_4=B2  logicinstr=X + W + Z  z_mux=C  xy_mux=A*B  w_mux=0  carry=0  dbl_ovrd=off  operand=+  x_mux=P  block_type=opmode
  Opmode3 : xbsIndex_r4/Opmode  device=DSP48E2  equ=P=PCIN+(A*B)  operation=Custom  inmode_0_3=D+A2  inmode_1_3=(D-A)*B  preaddinsel=A  amultsel=AD  bmultsel=B  inmode_0=A2  inmode_4=B2  logicinstr=X + W + Z  z_mux=PCIN  xy_mux=A*B  w_mux=0  carry=0  dbl_ovrd=off  operand=+  x_mux=P  block_type=opmode
  Reinterpret{,1..4,11,13} (7 alike) : xbsIndex_r4/Reinterpret  force_arith_type=on  arith_type="Signed  (2's comp)"  force_bin_pt=on  bin_pt=0  block_type=reinterpret
  Terminator : Terminator
  round1 : Subsystem
  out_real : Outport
  wires:
  Opmode3/1 -> DSP48E2 1/5
  Opmode2/1 -> "DSP48E2 "/5
  Delay1/1 -> DSP48E2 1/2
  Delay/1 -> DSP48E2 1/4
  round1/1(q) -> out_real/1
  Reinterpret13/1 -> round1/1(d)
  Reinterpret2/1 -> Convert3/1
  Convert7/1 -> "DSP48E2 "/4
  Reinterpret1/1 -> Convert2/1
  Constant3/1 -> "DSP48E2 "/3
  Reinterpret11/1 -> Convert7/1
  Reinterpret3/1 -> Convert4/1
  Convert3/1 -> DSP48E2 1/1
  Convert2/1 -> Delay1/1
  Convert4/1 -> Delay/1
  Reinterpret/1 -> Convert1/1
  Convert/1 -> "DSP48E2 "/1
  Convert1/1 -> "DSP48E2 "/2
  Reinterpret4/1 -> Convert/1
  DSP48E2 1/1 -> Reinterpret13/1
  "DSP48E2 "/1 -> Terminator/1
  "DSP48E2 "/2 -> DSP48E2 1/3
  Bi/1 -> Reinterpret11/1
  cos/1 -> Reinterpret/1
  Bq/1 -> Reinterpret3/1
  Ai/1 -> Reinterpret4/1
  Aq/1 -> Reinterpret2/1
  sin/1 -> Reinterpret1/1

== system pd_path_sg/resamp_mod/output_samp_E2_p0/up_sampi ==
  In1 : Inport
  Delay{1..7} (7 alike) : xbsIndex_r4/Delay  rst=off  infoeditControl=Selection of Reset will increase slice count due to use of real FFs and instead of SRLs  en=off  latency=2  reg_retiming=off  dbl_ovrd=off  block_type=delay
      settings: infoedit=Hardware notes: A delay line is a chain, each link of which is an SRL16 or SRL32 followed by a flip-flop.
  mult : Subsystem
  Out0 : Outport
  Out1 : Outport  Port=2
  wires:
  Delay7/1 -> Out0/1, mult/2(in2)
  Delay5/1 -> Delay6/1, mult/6(in6)
  Delay6/1 -> Delay7/1, mult/4(in4)
  In1/1 -> Delay1/1, mult/1(in1)
  Delay1/1 -> Delay2/1, mult/3(in3)
  Delay2/1 -> Delay3/1, mult/5(in5)
  mult/1(Out1) -> Out1/1
  Delay3/1 -> Delay4/1, mult/7(in7)
  Delay4/1 -> Delay5/1, mult/8(in8)

== system pd_path_sg/resamp_mod/output_samp_E2_p1/up_sampi ==
  In1 : Inport
  Delay{1..7} (7 alike) : xbsIndex_r4/Delay  rst=off  infoeditControl=Selection of Reset will increase slice count due to use of real FFs and instead of SRLs  en=off  latency=2  reg_retiming=off  dbl_ovrd=off  block_type=delay
      settings: infoedit=Hardware notes: A delay line is a chain, each link of which is an SRL16 or SRL32 followed by a flip-flop.
  mult : Subsystem
  Out0 : Outport
  Out1 : Outport  Port=2
  wires:
  Delay4/1 -> mult/8(in8), Delay5/1
  Delay3/1 -> mult/7(in7), Delay4/1
  mult/1(Out1) -> Out1/1
  Delay2/1 -> mult/5(in5), Delay3/1
  Delay1/1 -> mult/3(in3), Delay2/1
  In1/1 -> mult/1(in1), Delay1/1
  Delay6/1 -> mult/4(in4), Delay7/1
  Delay5/1 -> mult/6(in6), Delay6/1
  Delay7/1 -> mult/2(in2), Out0/1

== system pd_path_sg/resamp_mod/output_samp_E2_p2/up_sampi ==
  In1 : Inport
  Delay{1..7} (7 alike) : xbsIndex_r4/Delay  rst=off  infoeditControl=Selection of Reset will increase slice count due to use of real FFs and instead of SRLs  en=off  latency=2  reg_retiming=off  dbl_ovrd=off  block_type=delay
      settings: infoedit=Hardware notes: A delay line is a chain, each link of which is an SRL16 or SRL32 followed by a flip-flop.
  mult : Subsystem
  Out0 : Outport
  Out1 : Outport  Port=2
  wires:
  Delay7/1 -> Out0/1, mult/2(in2)
  Delay5/1 -> Delay6/1, mult/6(in6)
  Delay6/1 -> Delay7/1, mult/4(in4)
  In1/1 -> Delay1/1, mult/1(in1)
  Delay1/1 -> Delay2/1, mult/3(in3)
  Delay2/1 -> Delay3/1, mult/5(in5)
  mult/1(Out1) -> Out1/1
  Delay3/1 -> Delay4/1, mult/7(in7)
  Delay4/1 -> Delay5/1, mult/8(in8)

== system pd_path_sg/resamp_mod/output_samp_E2_p3/up_sampi ==
  In1 : Inport
  Delay{1..7} (7 alike) : xbsIndex_r4/Delay  rst=off  infoeditControl=Selection of Reset will increase slice count due to use of real FFs and instead of SRLs  en=off  latency=2  reg_retiming=off  dbl_ovrd=off  block_type=delay
      settings: infoedit=Hardware notes: A delay line is a chain, each link of which is an SRL16 or SRL32 followed by a flip-flop.
  mult : Subsystem
  Out0 : Outport
  Out1 : Outport  Port=2
  wires:
  Delay4/1 -> mult/8(in8), Delay5/1
  Delay3/1 -> mult/7(in7), Delay4/1
  mult/1(Out1) -> Out1/1
  Delay2/1 -> mult/5(in5), Delay3/1
  Delay1/1 -> mult/3(in3), Delay2/1
  In1/1 -> mult/1(in1), Delay1/1
  Delay6/1 -> mult/4(in4), Delay7/1
  Delay5/1 -> mult/6(in6), Delay6/1
  Delay7/1 -> mult/2(in2), Out0/1
